simulink model "example_algorithm_RLS"  (R2016a)
settings: Solver=VariableStepAuto  StartTime=0.0  StopTime=40  RelTol=1e-3
settings Model: Creator=mgreiff  LastModifiedBy=mgreiff

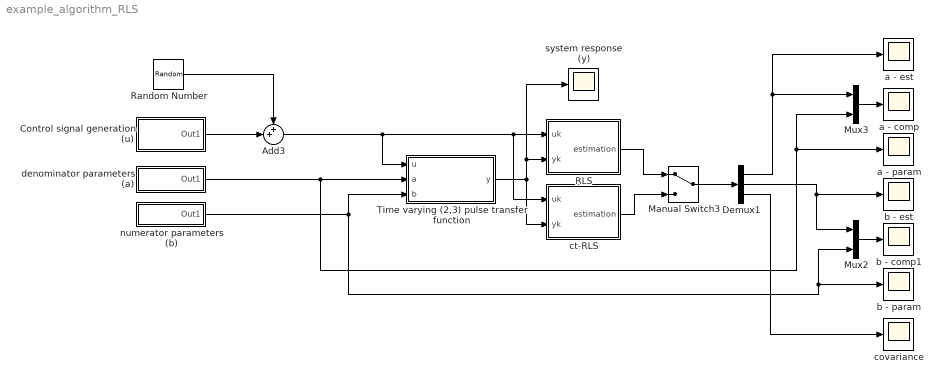
== system example_algorithm_RLS ==
  Add3 : Sum  Inputs=++|
  Control signal generation (u) : Subsystem
  Demux1 : Demux  Outputs=[2,2,1]
  Manual Switch3 : ManualSwitch
  Mux2 : Mux  Inputs=2
  Mux3 : Mux  Inputs=2
  RLS : Subsystem
  Random Number : RandomNumber  Variance=0.01  SampleTime=0.002
  Time varying (2,3) pulse transfer function : Subsystem
  a - comp : Scope
  a - est : Scope
  a - param : Scope
  b - comp1 : Scope
  b - est : Scope
  b - param : Scope
  covariance : Scope
  ct-RLS : Subsystem
  denominator parameters (a) : Subsystem
  numerator parameters (b) : Subsystem
  system response (y) : Scope
  wires:
  Random Number/1 -> Add3/1
  Demux1/1 -> Mux3/1, a - est/1
  Demux1/2 -> b - est/1, Mux2/1
  Mux2/1 -> b - comp1/1
  Mux3/1 -> a - comp/1
  Time varying (2,3) pulse transfer function/1(y) -> system response (y)/1, RLS/2(yk), ct-RLS/2(yk)
  Add3/1 -> Time varying (2,3) pulse transfer function/1(u), ct-RLS/1(uk), RLS/1(uk)
  Demux1/3 -> covariance/1
  ct-RLS/1(estimation) -> Manual Switch3/2
  Manual Switch3/1 -> Demux1/1
  RLS/1(estimation) -> Manual Switch3/1
  Control signal generation (u)/1(Out1) -> Add3/2
  denominator parameters (a)/1(Out1) -> a - param/1, Mux3/2, Time varying (2,3) pulse transfer function/2(a)
  numerator parameters (b)/1(Out1) -> Time varying (2,3) pulse transfer function/3(b), Mux2/2, b - param/1

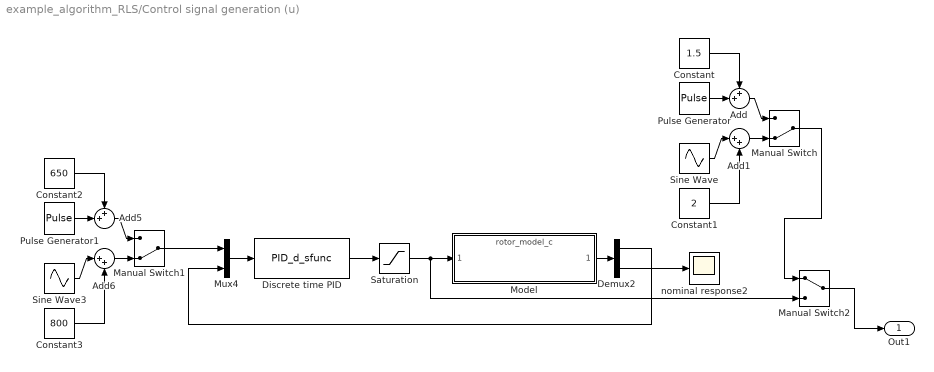
== system example_algorithm_RLS/Control signal generation (u) ==
  Add : Sum  Inputs=++|
  Add1 : Sum  Inputs=|++
  Add5 : Sum  Inputs=++|
  Add6 : Sum  Inputs=|++
  Constant : Constant  Value=1.5
  Constant1 : Constant  Value=2
  Constant2 : Constant  Value=650
  Constant3 : Constant  Value=800
  Demux2 : Demux  Outputs=[1,1]
  Discrete time PID : S-Function  FunctionName=PID_d_sfunc  Parameters=PIDparam  SFunctionDeploymentMode=off  EnableBusSupport=off
  Manual Switch : ManualSwitch  CurrentSetting=0
  Manual Switch1 : ManualSwitch  CurrentSetting=0
  Manual Switch2 : ManualSwitch
  Model : ModelReference  ModelNameDialog=rotor_model_c.slx  SimulationMode=Normal  ModelReferenceVersion=1.30
  Mux4 : Mux  Inputs=2
  Pulse Generator : DiscretePulseGenerator  PulseType=Time based  Amplitude=0.5  Period=4  PulseWidth=50
  Pulse Generator1 : DiscretePulseGenerator  PulseType=Time based  Amplitude=600  Period=4  PulseWidth=50
  Saturation : Saturate  UpperLimit=4.3  LowerLimit=0
  Sine Wave : Sin  Amplitude=-1  SampleTime=0
  Sine Wave3 : Sin  Amplitude=300  SampleTime=0
  nominal response2 : Scope
  Out1 : Outport
  wires:
  Constant/1 -> Add/1
  Pulse Generator/1 -> Add/2
  Add/1 -> Manual Switch/1
  Sine Wave/1 -> Add1/1
  Constant1/1 -> Add1/2
  Add1/1 -> Manual Switch/2
  Discrete time PID/1 -> Saturation/1
  Pulse Generator1/1 -> Add5/2
  Constant2/1 -> Add5/1
  Add5/1 -> Manual Switch1/1
  Sine Wave3/1 -> Add6/1
  Add6/1 -> Manual Switch1/2
  Manual Switch1/1 -> Mux4/1
  Constant3/1 -> Add6/2
  Mux4/1 -> Discrete time PID/1
  Model/1 -> Demux2/1
  Demux2/2 -> nominal response2/1
  Demux2/1 -> Mux4/2
  Manual Switch/1 -> Manual Switch2/1
  Manual Switch2/1 -> Out1/1
  Saturation/1 -> Manual Switch2/2, Model/1

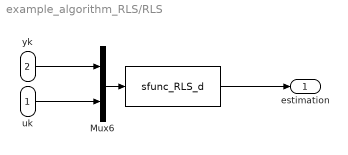
== system example_algorithm_RLS/RLS ==
  uk : Inport
  yk : Inport  Port=2
  "   " : S-Function  FunctionName=sfunc_RLS_d  Parameters=RLSparam  SFunctionDeploymentMode=off  EnableBusSupport=off
  Mux6 : Mux  Inputs=2
  estimation : Outport
  wires:
  yk/1 -> Mux6/1
  uk/1 -> Mux6/2
  "   "/1 -> estimation/1
  Mux6/1 -> "   "/1

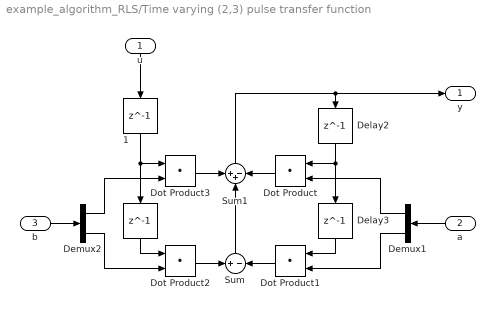
== system example_algorithm_RLS/Time varying (2,3) pulse transfer function ==
  u : Inport
  a : Inport  Port=2
  b : Inport  Port=3
  "  " : Delay  DelayLength=1  InitialCondition=0  SampleTime=0.002
  "  1" : Delay  DelayLength=1  InitialCondition=0  SampleTime=0.002
  Delay2 : Delay  DelayLength=1  InitialCondition=0  SampleTime=0.002
  Delay3 : Delay  DelayLength=1  InitialCondition=0  SampleTime=0.002
  Demux1 : Demux  Outputs=[1,1]
  Demux2 : Demux  Outputs=[1,1]
  Dot Product{,1..3} (4 alike) : DotProduct  InputSameDT=on  OutDataTypeStr=Inherit: Inherit via internal rule
  Sum : Sum  Inputs=+|-
  Sum1 : Sum  Inputs=++-
  y : Outport
  wires:
  Dot Product2/1 -> Sum/1
  Demux2/2 -> Dot Product2/2
  Dot Product1/1 -> Sum/2
  Delay3/1 -> Dot Product1/1
  "  "/1 -> Dot Product2/1
  Dot Product/1 -> Sum1/3
  Delay2/1 -> Dot Product/1, Delay3/1
  Demux1/2 -> Dot Product1/2
  Demux1/1 -> Dot Product/2
  u/1 -> "  1"/1
  "  1"/1 -> Dot Product3/1, "  "/1
  Sum1/1 -> Delay2/1, y/1
  Dot Product3/1 -> Sum1/1
  Sum/1 -> Sum1/2
  a/1 -> Demux1/1
  Demux2/1 -> Dot Product3/2
  b/1 -> Demux2/1

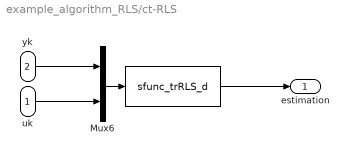
== system example_algorithm_RLS/ct-RLS ==
  uk : Inport
  yk : Inport  Port=2
  "   " : S-Function  FunctionName=sfunc_trRLS_d  Parameters=trRLSparam  SFunctionDeploymentMode=off  EnableBusSupport=off
  Mux6 : Mux  Inputs=2
  estimation : Outport
  wires:
  yk/1 -> Mux6/1
  uk/1 -> Mux6/2
  "   "/1 -> estimation/1
  Mux6/1 -> "   "/1

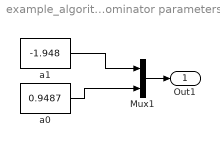
== system example_algorithm_RLS/denominator parameters (a) ==
  Mux1 : Mux  Inputs=2
  a0 : Constant  Value=0.9487
  a1 : Constant  Value=-1.948
  Out1 : Outport
  wires:
  Mux1/1 -> Out1/1
  a0/1 -> Mux1/2
  a1/1 -> Mux1/1

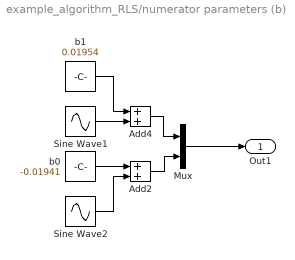
== system example_algorithm_RLS/numerator parameters (b) ==
  Add2 : Sum
  Add4 : Sum
  Mux : Mux  Inputs=2
  Sine Wave1 : Sin  Amplitude=0.01  Frequency=0.2  SampleTime=0
  Sine Wave2 : Sin  Amplitude=0.005  Frequency=0.4  SampleTime=0
  b0 : Constant  Value=-0.01941
  b1 : Constant  Value=0.01954
  Out1 : Outport
  wires:
  Add4/1 -> Mux/1
  Mux/1 -> Out1/1
  Add2/1 -> Mux/2
  b0/1 -> Add2/1
  b1/1 -> Add4/1
  Sine Wave2/1 -> Add2/2
  Sine Wave1/1 -> Add4/2
